simulink model "MicrogridControl"  (R2025b)
settings: Solver=VariableStepAuto  StartTime=0.0  StopTime=8  FixedStep=Ts  RelTol=1e-3
PreLoadFcn:
  | NormalOperation;
  | MicrogridControlParam;
undefined symbols (not defined in the file): base, bessModeInitial, bessSystem, bessVoltage, breakerStatus, DiscIntNeverNeededParam, ee_sli_rtmsupport, event, gcbh, generator, gflInverter, gfmInverter, Inertia, lineInductance, lineResistance, machine, plannedIsland, pmsm, powerLimit, powerQuality, PV, PVInverter, ref, resync, solar, solarInsolationChange, systemFrequency, Ts, windController, windSystem, windTurbine
libraries: nesl_utility x234, ee_lib x174, fl_lib x143, eeGeneralControl x137, simulink x78, eeTransforms x47, slpidlib x23, nesl_utility_internal x12, eePwmGenerator x9, eeSinusoidalMeasurementV2 x9, custom_lib x7, batteryecm_lib x6
(part 2 of 25)

== system MicrogridControl/BESS ==
  BusElementIn : Inport  PortName=InBus  Element=activePower
  BusElementIn1 : Inport  PortName=InBus  Element=reactivePower
  BusElementIn2 : Inport  PortName=InBus  Element=voltage
  BusElementIn3 : Inport  PortName=InBus  Element=frequency
  BusElementIn4 : Inport  PortName=InBus  Element=mode
  BusElementIn5 : Inport  PortName=InBus  Element=activePowerBESS1
  BESS Integrated : Subsystem  Variant=on  VariantControlMode=label  LabelModeActiveChoice=Detailed  mask(Battery Energy Storage System (BESS)){fidelity=Detailed, bessController=Grid Forming, plantRating=bessSystem.plantRating/2, Vac=bessSystem.Vac, frequency=bessSystem.frequency, iMaxPU=bessSystem.iMaxPU, efficiency=bessSystem.converterEfficiency, baseVoltageDC=bessSystem.Vdc, filterInductance=bessSystem.filterInductance, filterResistance=bessSystem.filterResistance, maxSOC=bessSystem.maxSOC, minSOC=bessSystem.minSOC, converterFidelity=Average, fSw=bessSystem.switchingFrequency, activeDroop=bessSystem.activeDroop, reactiveDroop=bessSystem.reactiveDroop, maxSOCGFM=0.95, minSOCGFM=0.1, initialSOC=0.9, capacityType=Infinite, capacity=1000}
      mask prompts: fidelity "Modeling Option"; bessController "Operating Mode"; plantRating "BESS Rating (kW)"; Vac "Rated AC side voltage (phase-phase RMS) (V)"; frequency "Rated electrical frequency at AC side (Hz)"; iMaxPU "Maximum converter current (pu)"; efficiency "Converter Efficiency (%)"; baseVoltageDC "Voltage on DC side (V)"; filterInductance "Filter inductance (H)"; filterResistance "Filter series resistance (Ohm)"; maxSOC "Maximum  operating SOC"; minSOC "Minimum  operating SOC"; converterFidelity "Converter Fidelity"; fSw "Switching Frequency (kHz)"; activeDroop "Active droop"; reactiveDroop "Reactive droop"; maxSOCGFM "Maximum  operating SOC"; minSOCGFM "Minimum  operating SOC"; initialSOC "Initial SOC"; capacityType "Battery charge capacity"; capacity "Battery capacity (Ah)"
      mask help:
      | This block represents a flexible BESS that can be configured for different operational modes and modeling fidelities. It supports Grid-Following (GFL) and Grid-Forming (GFM) control strategies, along with two fidelity levels:
      |
      | Detailed – captures dynamic control loops and converter behavior for accurate transient analysis.
      | Simplified – optimized for faster simulations while preserving essential system characteristics.
      settings: CopyFcn=set_param(gcbh,'LinkStatus','none');
      mask Help: web('BESS.html')
      mask TypeOptions fidelity: Detailed | Simplified
      mask Callback fidelity:
      | component.mask.fidelitySelection;
      |     fidelity = get_param(gcb,'fidelity');
      |     mode = get_param(gcb,'bessController');
      |     maskObj = Simulink.Mask.get(gcb);
      |     allNames = {maskObj.Parameters.Name};
      |     effIdx = find(strcmp(allNames, 'efficiency'));
      |     tabGFL = maskObj.getDialogControl('cellSimplified');
      |     tabGFM = maskObj.getDialogControl('cellSimplifiedGFM');
      |     if strcmp(fidelity,'Simplified')
      |         maskObj.Parameters(effIdx).Visible = 'on';
      |         if strcmp(mode,'Grid Following')
      |             tabGFL.Visible = 'on';
      |             tabGFM.Visible = 'off';
      |         else
      |             tabGFL.Visible = 'off';
      |             tabGFM.Visible = 'on';
      |         end
      |     else
      |         maskObj.Parameters(effIdx).Visible = 'off';
      |         tabGFL.Visible = 'off';
      |         tabGFM.Visible = 'off';
      |     end
      mask TypeOptions bessController: Grid Following | Grid Forming
      mask Callback bessController:
      | fidelity = get_param(gcb,'fidelity');
      | mode = get_param(gcb,'bessController');
      | if strcmp(fidelity,'Detailed')
      |     component.mask.setBESSController;
      | else
      |     blockPath = [gcb,'/','Simplified'];
      |     component.mask.setBESSController(blockPath);
      | end
      | maskObj = Simulink.Mask.get(gcb);
      | tabGFL = maskObj.getDialogControl('cellSimplified');
      | tabGFM = maskObj.getDialogControl('cellSimplifiedGFM');
      | if strcmp(fidelity,'Simplified')
      |     if strcmp(mode,'Grid Following')
      |         tabGFL.Visible = 'on';
      |         tabGFM.Visible = 'off';
      |     else
      |         tabGFL.Visible = 'off';
      |         tabGFM.Visible = 'on';
      |     end
      | else
      |     tabGFL.Visible = 'off';
      |     tabGFM.Visible = 'off';
      | end
      mask TypeOptions converterFidelity: Detailed/BESS Plant/converterFidelity
      mask Callback converterFidelity:
      | blockPath = [gcb,'/','Detailed','/','BESS Plant','/','Converter'];
      | component.mask.converterFidelity(blockPath);
      mask TypeOptions fSw: Detailed/PV Plant & Controller/PV Plant/fSw
      mask TypeOptions initialSOC: Simplified/Grid Forming/initialSOC
      mask TypeOptions capacityType: Simplified/Grid Forming/capacityType
      mask Callback capacityType: component.mask.configureBatteryCapacity;
      mask TypeOptions capacity: Simplified/Grid Forming/capacity
      mask DialogControl generalDetailed Prompt: General
      mask DialogControl cellDetailed Prompt: Battery
      mask DialogControl configureBattery Prompt: Edit battery parameters
      mask DialogControl configureBattery Callback:
      | blockPath = [gcb,'/','Detailed','/','BESS Plant','/','Battery'] ;
      |     component.mask.openBlock(blockPath);
      mask DialogControl controllerDetailed Prompt: BESS Controller
      mask DialogControl configureBESSController Prompt: Edit BESS Controller
      mask DialogControl configureBESSController Callback:
      | controllerType = get_param(gcb,'bessController');
      |     blockPath = [gcb,'/','Detailed','/','BESS Controller','/',controllerType];
      |     component.mask.openBlock(blockPath);
      mask DialogControl cellSimplified Prompt: Battery
      mask DialogControl configureBatterySimplified Prompt: Edit battery parameters
      mask DialogControl configureBatterySimplified Callback:
      | mode = get_param(gcb,'bessController');
      |     blockPath = [gcb,'/','Simplified','/',mode,'/','Battery'] ;
      |     if strcmp(mode,'Grid Following')
      |         component.mask.openBlock(blockPath);
      |     end
      mask DialogControl converter Prompt: Converter
      mask DialogControl editConverter Prompt: Edit converter parameters
      mask DialogControl editConverter Callback:
      | converterFidelity = get_param(gcb,'converterFidelity');
      | blockPath = [gcb,'/','Detailed','/','BESS Plant','/','Converter','/',converterFidelity,'/','Converter'];
      | component.mask.openBlock(blockPath);
      mask DialogControl cellSimplifiedGFM Prompt: Battery
      mask Display: image('battery_detailed.png');
  BESS Integrated1 : Subsystem  Variant=on  VariantControlMode=label  LabelModeActiveChoice=Detailed  mask(Battery Energy Storage System (BESS)){fidelity=Detailed, bessController=Grid Forming, plantRating=bessSystem.plantRating/2, Vac=bessSystem.Vac, frequency=bessSystem.frequency, iMaxPU=bessSystem.iMaxPU, efficiency=bessSystem.converterEfficiency, baseVoltageDC=bessSystem.Vdc, filterInductance=bessSystem.filterInductance, filterResistance=bessSystem.filterResistance, maxSOC=bessSystem.maxSOC, minSOC=bessSystem.minSOC, converterFidelity=Average, fSw=bessSystem.switchingFrequency, activeDroop=bessSystem.activeDroop, reactiveDroop=bessSystem.reactiveDroop, maxSOCGFM=0.95, minSOCGFM=0.1, initialSOC=0.9, capacityType=Infinite, capacity=1000}
      mask prompts: fidelity "Modeling Option"; bessController "Operating Mode"; plantRating "BESS Rating (kW)"; Vac "Rated AC side voltage (phase-phase RMS) (V)"; frequency "Rated electrical frequency at AC side (Hz)"; iMaxPU "Maximum converter current (pu)"; efficiency "Converter Efficiency (%)"; baseVoltageDC "Voltage on DC side (V)"; filterInductance "Filter inductance (H)"; filterResistance "Filter series resistance (Ohm)"; maxSOC "Maximum  operating SOC"; minSOC "Minimum  operating SOC"; converterFidelity "Converter Fidelity"; fSw "Switching Frequency (kHz)"; activeDroop "Active droop"; reactiveDroop "Reactive droop"; maxSOCGFM "Maximum  operating SOC"; minSOCGFM "Minimum  operating SOC"; initialSOC "Initial SOC"; capacityType "Battery charge capacity"; capacity "Battery capacity (Ah)"
      mask help:
      | This block represents a flexible BESS that can be configured for different operational modes and modeling fidelities. It supports Grid-Following (GFL) and Grid-Forming (GFM) control strategies, along with two fidelity levels:
      |
      | Detailed – captures dynamic control loops and converter behavior for accurate transient analysis.
      | Simplified – optimized for faster simulations while preserving essential system characteristics.
      settings: CopyFcn=set_param(gcbh,'LinkStatus','none');
      mask Help: web('BESS.html')
      mask TypeOptions fidelity: Detailed | Simplified
      mask Callback fidelity:
      | component.mask.fidelitySelection;
      |     fidelity = get_param(gcb,'fidelity');
      |     mode = get_param(gcb,'bessController');
      |     maskObj = Simulink.Mask.get(gcb);
      |     allNames = {maskObj.Parameters.Name};
      |     effIdx = find(strcmp(allNames, 'efficiency'));
      |     tabGFL = maskObj.getDialogControl('cellSimplified');
      |     tabGFM = maskObj.getDialogControl('cellSimplifiedGFM');
      |     if strcmp(fidelity,'Simplified')
      |         maskObj.Parameters(effIdx).Visible = 'on';
      |         if strcmp(mode,'Grid Following')
      |             tabGFL.Visible = 'on';
      |             tabGFM.Visible = 'off';
      |         else
      |             tabGFL.Visible = 'off';
      |             tabGFM.Visible = 'on';
      |         end
      |     else
      |         maskObj.Parameters(effIdx).Visible = 'off';
      |         tabGFL.Visible = 'off';
      |         tabGFM.Visible = 'off';
      |     end
      mask TypeOptions bessController: Grid Following | Grid Forming
      mask Callback bessController:
      | fidelity = get_param(gcb,'fidelity');
      | mode = get_param(gcb,'bessController');
      | if strcmp(fidelity,'Detailed')
      |     component.mask.setBESSController;
      | else
      |     blockPath = [gcb,'/','Simplified'];
      |     component.mask.setBESSController(blockPath);
      | end
      | maskObj = Simulink.Mask.get(gcb);
      | tabGFL = maskObj.getDialogControl('cellSimplified');
      | tabGFM = maskObj.getDialogControl('cellSimplifiedGFM');
      | if strcmp(fidelity,'Simplified')
      |     if strcmp(mode,'Grid Following')
      |         tabGFL.Visible = 'on';
      |         tabGFM.Visible = 'off';
      |     else
      |         tabGFL.Visible = 'off';
      |         tabGFM.Visible = 'on';
      |     end
      | else
      |     tabGFL.Visible = 'off';
      |     tabGFM.Visible = 'off';
      | end
      mask TypeOptions converterFidelity: Detailed/BESS Plant/converterFidelity
      mask Callback converterFidelity:
      | blockPath = [gcb,'/','Detailed','/','BESS Plant','/','Converter'];
      | component.mask.converterFidelity(blockPath);
      mask TypeOptions fSw: Detailed/PV Plant & Controller/PV Plant/fSw
      mask TypeOptions initialSOC: Simplified/Grid Forming/initialSOC
      mask TypeOptions capacityType: Simplified/Grid Forming/capacityType
      mask Callback capacityType: component.mask.configureBatteryCapacity;
      mask TypeOptions capacity: Simplified/Grid Forming/capacity
      mask DialogControl generalDetailed Prompt: General
      mask DialogControl cellDetailed Prompt: Battery
      mask DialogControl configureBattery Prompt: Edit battery parameters
      mask DialogControl configureBattery Callback:
      | blockPath = [gcb,'/','Detailed','/','BESS Plant','/','Battery'] ;
      |     component.mask.openBlock(blockPath);
      mask DialogControl controllerDetailed Prompt: BESS Controller
      mask DialogControl configureBESSController Prompt: Edit BESS Controller
      mask DialogControl configureBESSController Callback:
      | controllerType = get_param(gcb,'bessController');
      |     blockPath = [gcb,'/','Detailed','/','BESS Controller','/',controllerType];
      |     component.mask.openBlock(blockPath);
      mask DialogControl cellSimplified Prompt: Battery
      mask DialogControl configureBatterySimplified Prompt: Edit battery parameters
      mask DialogControl configureBatterySimplified Callback:
      | mode = get_param(gcb,'bessController');
      |     blockPath = [gcb,'/','Simplified','/',mode,'/','Battery'] ;
      |     if strcmp(mode,'Grid Following')
      |         component.mask.openBlock(blockPath);
      |     end
      mask DialogControl converter Prompt: Converter
      mask DialogControl editConverter Prompt: Edit converter parameters
      mask DialogControl editConverter Callback:
      | converterFidelity = get_param(gcb,'converterFidelity');
      | blockPath = [gcb,'/','Detailed','/','BESS Plant','/','Converter','/',converterFidelity,'/','Converter'];
      | component.mask.openBlock(blockPath);
      mask DialogControl cellSimplifiedGFM Prompt: Battery
      mask Display: image('battery_detailed.png');
  BESS Integrated3 : Subsystem  Variant=on  VariantControlMode=label  LabelModeActiveChoice=Detailed  mask(Battery Energy Storage System (BESS)){fidelity=Detailed, bessController=Grid Forming, plantRating=bessSystem.plantRating*1.5, Vac=bessSystem.Vac, frequency=bessSystem.frequency, iMaxPU=bessSystem.iMaxPU, efficiency=bessSystem.converterEfficiency, baseVoltageDC=bessSystem.Vdc, filterInductance=bessSystem.filterInductance, filterResistance=bessSystem.filterResistance, maxSOC=bessSystem.maxSOC, minSOC=bessSystem.minSOC, converterFidelity=Average, fSw=bessSystem.switchingFrequency, activeDroop=bessSystem.activeDroop, reactiveDroop=bessSystem.reactiveDroop, maxSOCGFM=0.95, minSOCGFM=0.1, initialSOC=0.9, capacityType=Infinite, capacity=1000}
      mask prompts: fidelity "Modeling Option"; bessController "Operating Mode"; plantRating "BESS Rating (kW)"; Vac "Rated AC side voltage (phase-phase RMS) (V)"; frequency "Rated electrical frequency at AC side (Hz)"; iMaxPU "Maximum converter current (pu)"; efficiency "Converter Efficiency (%)"; baseVoltageDC "Voltage on DC side (V)"; filterInductance "Filter inductance (H)"; filterResistance "Filter series resistance (Ohm)"; maxSOC "Maximum  operating SOC"; minSOC "Minimum  operating SOC"; converterFidelity "Converter Fidelity"; fSw "Switching Frequency (kHz)"; activeDroop "Active droop"; reactiveDroop "Reactive droop"; maxSOCGFM "Maximum  operating SOC"; minSOCGFM "Minimum  operating SOC"; initialSOC "Initial SOC"; capacityType "Battery charge capacity"; capacity "Battery capacity (Ah)"
      mask help:
      | This block represents a flexible BESS that can be configured for different operational modes and modeling fidelities. It supports Grid-Following (GFL) and Grid-Forming (GFM) control strategies, along with two fidelity levels:
      |
      | Detailed – captures dynamic control loops and converter behavior for accurate transient analysis.
      | Simplified – optimized for faster simulations while preserving essential system characteristics.
      settings: CopyFcn=set_param(gcbh,'LinkStatus','none');
      mask Help: web('BESS.html')
      mask TypeOptions fidelity: Detailed | Simplified
      mask Callback fidelity:
      | component.mask.fidelitySelection;
      |     fidelity = get_param(gcb,'fidelity');
      |     mode = get_param(gcb,'bessController');
      |     maskObj = Simulink.Mask.get(gcb);
      |     allNames = {maskObj.Parameters.Name};
      |     effIdx = find(strcmp(allNames, 'efficiency'));
      |     tabGFL = maskObj.getDialogControl('cellSimplified');
      |     tabGFM = maskObj.getDialogControl('cellSimplifiedGFM');
      |     if strcmp(fidelity,'Simplified')
      |         maskObj.Parameters(effIdx).Visible = 'on';
      |         if strcmp(mode,'Grid Following')
      |             tabGFL.Visible = 'on';
      |             tabGFM.Visible = 'off';
      |         else
      |             tabGFL.Visible = 'off';
      |             tabGFM.Visible = 'on';
      |         end
      |     else
      |         maskObj.Parameters(effIdx).Visible = 'off';
      |         tabGFL.Visible = 'off';
      |         tabGFM.Visible = 'off';
      |     end
      mask TypeOptions bessController: Grid Following | Grid Forming
      mask Callback bessController:
      | fidelity = get_param(gcb,'fidelity');
      | mode = get_param(gcb,'bessController');
      | if strcmp(fidelity,'Detailed')
      |     component.mask.setBESSController;
      | else
      |     blockPath = [gcb,'/','Simplified'];
      |     component.mask.setBESSController(blockPath);
      | end
      | maskObj = Simulink.Mask.get(gcb);
      | tabGFL = maskObj.getDialogControl('cellSimplified');
      | tabGFM = maskObj.getDialogControl('cellSimplifiedGFM');
      | if strcmp(fidelity,'Simplified')
      |     if strcmp(mode,'Grid Following')
      |         tabGFL.Visible = 'on';
      |         tabGFM.Visible = 'off';
      |     else
      |         tabGFL.Visible = 'off';
      |         tabGFM.Visible = 'on';
      |     end
      | else
      |     tabGFL.Visible = 'off';
      |     tabGFM.Visible = 'off';
      | end
      mask TypeOptions converterFidelity: Detailed/BESS Plant/converterFidelity
      mask Callback converterFidelity:
      | blockPath = [gcb,'/','Detailed','/','BESS Plant','/','Converter'];
      | component.mask.converterFidelity(blockPath);
      mask TypeOptions fSw: Detailed/PV Plant & Controller/PV Plant/fSw
      mask TypeOptions initialSOC: Simplified/Grid Forming/initialSOC
      mask TypeOptions capacityType: Simplified/Grid Forming/capacityType
      mask Callback capacityType: component.mask.configureBatteryCapacity;
      mask TypeOptions capacity: Simplified/Grid Forming/capacity
      mask DialogControl generalDetailed Prompt: General
      mask DialogControl cellDetailed Prompt: Battery
      mask DialogControl configureBattery Prompt: Edit battery parameters
      mask DialogControl configureBattery Callback:
      | blockPath = [gcb,'/','Detailed','/','BESS Plant','/','Battery'] ;
      |     component.mask.openBlock(blockPath);
      mask DialogControl controllerDetailed Prompt: BESS Controller
      mask DialogControl configureBESSController Prompt: Edit BESS Controller
      mask DialogControl configureBESSController Callback:
      | controllerType = get_param(gcb,'bessController');
      |     blockPath = [gcb,'/','Detailed','/','BESS Controller','/',controllerType];
      |     component.mask.openBlock(blockPath);
      mask DialogControl cellSimplified Prompt: Battery
      mask DialogControl configureBatterySimplified Prompt: Edit battery parameters
      mask DialogControl configureBatterySimplified Callback:
      | mode = get_param(gcb,'bessController');
      |     blockPath = [gcb,'/','Simplified','/',mode,'/','Battery'] ;
      |     if strcmp(mode,'Grid Following')
      |         component.mask.openBlock(blockPath);
      |     end
      mask DialogControl converter Prompt: Converter
      mask DialogControl editConverter Prompt: Edit converter parameters
      mask DialogControl editConverter Callback:
      | converterFidelity = get_param(gcb,'converterFidelity');
      | blockPath = [gcb,'/','Detailed','/','BESS Plant','/','Converter','/',converterFidelity,'/','Converter'];
      | component.mask.openBlock(blockPath);
      mask DialogControl cellSimplifiedGFM Prompt: Battery
      mask Display: image('battery_detailed.png');
  Bus Selector : BusSelector  OutputSignals=activePower,reactivePower
  Bus Selector1 : BusSelector  OutputSignals=activePower,reactivePower
  Bus Selector2 : BusSelector  OutputSignals=activePower,reactivePower
  Constant : Constant
  Constant1 : Constant
  Constant3 : Constant  Value=ref.QBESS1MW
  Constant4 : Constant
  Constant5 : Constant  Value=0
  Constant7 : Constant  Value=0
  Delay : Delay  DelayLength=100  InitialCondition=bessModeInitial  InputProcessing=Columns as channels (frame based)
  Gain1 : Gain
  Rate Transition : RateTransition  Deterministic=off  OutPortSampleTime=Ts
  Rate Transition1 : RateTransition  OutPortSampleTime=Ts
  Rate Transition2 : RateTransition  Deterministic=off  OutPortSampleTime=Ts
  Rate Transition3 : RateTransition  OutPortSampleTime=Ts
  Scope2 : Scope  NumInputPorts=2
      settings: ActiveDisplayYMinimum=-0.28740391792348163  ActiveDisplayYMaximum=0.22078217074426204  DataLoggingVariableName=ScopeData53
  Scope3 : Scope  NumInputPorts=2
      settings: ActiveDisplayYMinimum=-0.88278351750877571  ActiveDisplayYMaximum=1.6943513796670802  DataLoggingVariableName=ScopeData54
  Scope4 : Scope  NumInputPorts=2
      settings: ActiveDisplayYMinimum=-0.88286408189414312  ActiveDisplayYMaximum=1.6939099105793236  DataLoggingVariableName=ScopeData55
  Transformer : Subsystem  Variant=on  VariantControlMode=label  LabelModeActiveChoice=Detailed  mask{fidelity=Detailed}
      mask prompts: fidelity "Modeling Option"
      mask TypeOptions fidelity: Detailed | Simplified
      mask Callback fidelity:
      | choice = get_param(gcb,'fidelity');
      | switch choice
      |     case 'Detailed'
      |         set_param(gcb, 'LabelModeActiveChoice', 'Detailed');
      |     case 'Simplified'
      |          set_param(gcb, 'LabelModeActiveChoice', 'Simplified');
      |     otherwise
      |         disp('Choose proper variant');
      | end
  Transformer1 : Subsystem  Variant=on  VariantControlMode=label  LabelModeActiveChoice=Detailed  mask{fidelity=Detailed}
      mask prompts: fidelity "Modeling Option"
      mask TypeOptions fidelity: Detailed | Simplified
      mask Callback fidelity:
      | choice = get_param(gcb,'fidelity');
      | switch choice
      |     case 'Detailed'
      |         set_param(gcb, 'LabelModeActiveChoice', 'Detailed');
      |     case 'Simplified'
      |          set_param(gcb, 'LabelModeActiveChoice', 'Simplified');
      |     otherwise
      |         disp('Choose proper variant');
      | end
  Transformer3 : Subsystem  Variant=on  VariantControlMode=label  LabelModeActiveChoice=Detailed  mask{fidelity=Detailed}
      mask prompts: fidelity "Modeling Option"
      mask TypeOptions fidelity: Detailed | Simplified
      mask Callback fidelity:
      | choice = get_param(gcb,'fidelity');
      | switch choice
      |     case 'Detailed'
      |         set_param(gcb, 'LabelModeActiveChoice', 'Detailed');
      |     case 'Simplified'
      |          set_param(gcb, 'LabelModeActiveChoice', 'Simplified');
      |     otherwise
      |         disp('Choose proper variant');
      | end
  ~ : PMIOPort  Side=Left
  wires:
  Constant1/1 -> BESS Integrated/2(FRef), BESS Integrated1/2(FRef)
  Constant/1 -> BESS Integrated/1(VRef), BESS Integrated1/1(VRef)
  Constant5/1 -> BESS Integrated/6(Reset), BESS Integrated1/6(Reset)
  Constant3/1 -> BESS Integrated/4(QRef), BESS Integrated1/4(QRef)
  BusElementIn/1 -> Rate Transition/1
  BusElementIn1/1 -> Rate Transition1/1
  BusElementIn2/1 -> Rate Transition2/1
  BusElementIn3/1 -> Rate Transition3/1
  Rate Transition2/1 -> BESS Integrated3/1(VRef)
  Rate Transition3/1 -> BESS Integrated3/2(FRef)
  BusElementIn4/1 -> Delay/1
  Constant7/1 -> BESS Integrated3/6(Reset)
  Delay/1 -> Gain1/1
  BESS Integrated3/1(Meas) -> Bus Selector/1
  Bus Selector/1 -> Scope2/1  "<activePower>"
  Bus Selector/2 -> Scope2/2  "<reactivePower>"
  BESS Integrated1/1(Meas) -> Bus Selector1/1
  BESS Integrated/1(Meas) -> Bus Selector2/1
  Bus Selector1/2 -> Scope3/2  "<reactivePower>"
  Bus Selector1/1 -> Scope3/1  "<activePower>"
  Rate Transition/1 -> BESS Integrated3/3(PRef)
  Rate Transition1/1 -> BESS Integrated3/4(QRef)
  Bus Selector2/1 -> Scope4/1  "<activePower>"
  Bus Selector2/2 -> Scope4/2  "<reactivePower>"
  Constant4/1 -> BESS Integrated1/5(Mode), BESS Integrated/5(Mode)
  BusElementIn5/1 -> BESS Integrated1/3(PRef), BESS Integrated/3(PRef)
  Gain1/1 -> BESS Integrated3/5(Mode)
  connections:
  BESS Integrated/RConn1 -- Transformer/LConn1
  BESS Integrated1/RConn1 -- Transformer1/LConn1
  BESS Integrated3/RConn1 -- Transformer3/LConn1
  Transformer1/RConn1 -- Transformer3/RConn1 -- Transformer/RConn1 -- ~/RConn1

== system MicrogridControl/Control Room ==
  Constant1 : Constant  Value=ref.PBESS3MW%0.4  SampleTime=-1
  Constant2 : Constant  Value=0
  Constant3 : Constant  SampleTime=-1
  Constant4 : Constant  Value=ref.QBESS3MW%0.2  SampleTime=-1
  Constant5 : Constant  SampleTime=-1
  Constant6 : Constant  Value=0
  Constant7 : Constant  Commented=on  Value=0.45  SampleTime=-1
  Constant8 : Constant  Commented=on  Value=0.2  SampleTime=-1
  Data Type Conversion{3,5..7} (4 alike) : DataTypeConversion  OutDataTypeStr=boolean  SaturateOnIntegerOverflow=off  RndMeth=Floor
  PlannedIslandCommand : Step  Time=event.plannedIslanding  SampleTime=Ts
  Resynch Command : Step  Time=event.resynchronization  SampleTime=Ts
  Resynch Command1 : Step  Time=event.resynchronization  After=0  SampleTime=Ts
  Step13 : Step  Time=1000  After=-1  SampleTime=Ts
  Step16 : Step  Time=1000  SampleTime=Ts
  Step8 : Step  Time=1000  SampleTime=Ts
  Sum : Sum  Inputs=|++
  Out Bus Element5 : Outport  PortName=CtrlRm  Element=blackStart
  Out Bus Element4 : Outport  PortName=CtrlRm  Element=blackStartReset
  Out Bus Element19 : Outport  PortName=CtrlRm  Element=PowerCmd
  Out Bus Element20 : Outport  PortName=CtrlRm  Element=unplannedIslanding
  Out Bus Element22 : Outport  PortName=CtrlRm  Element=BESSReactivePower
  Out Bus Element18 : Outport  PortName=CtrlRm  Element=Resync
  Out Bus Element3 : Outport  PortName=CtrlRm  Element=FRef
  Out Bus Element6 : Outport  PortName=CtrlRm  Element=plannedIslanding
  Out Bus Element1 : Outport  PortName=CtrlRm  Element=QRef
  Out Bus Element2 : Outport  PortName=CtrlRm  Element=VRef
  Out Bus Element : Outport  PortName=CtrlRm  Element=PRef
  BusElementOut : Outport  PortName=CtrlRm  Element=BRKcontrol
  wires:
  Constant4/1 -> Out Bus Element1/1  "Reactive Power Setpoint"
  Data Type Conversion6/1 -> Out Bus Element18/1
  Step13/1 -> Sum/1  "Blackstart"
  Data Type Conversion7/1 -> Out Bus Element5/1
  Data Type Conversion3/1 -> Out Bus Element6/1
  Step8/1 -> Data Type Conversion7/1, Sum/2  "Blackstart"
  Constant5/1 -> Out Bus Element3/1  "Frequency Setpoint"
  Constant6/1 -> Out Bus Element22/1
  PlannedIslandCommand/1 -> Data Type Conversion3/1  "Planned Island_Command2"
  Resynch Command1/1 -> Out Bus Element19/1  "Power Tracking Command"
  Resynch Command/1 -> Data Type Conversion6/1  "Resynch_Command2"
  Constant1/1 -> Out Bus Element/1  "Active Power setpoint"
  Sum/1 -> Out Bus Element4/1
  Constant3/1 -> Out Bus Element2/1  "Voltage Setpoint"
  Step16/1 -> Data Type Conversion5/1  "VF mode"
  Data Type Conversion5/1 -> Out Bus Element20/1
  Constant2/1 -> BusElementOut/1

== system MicrogridControl/Domestic Load ==
  Circuit Breaker : Subsystem
  Electrical Reference1 : fl_lib/Electrical/Electrical Elements/Electrical Reference
  Electrical Reference2 : fl_lib/Electrical/Electrical Elements/Electrical Reference
  Load1 : ee_lib/Passive/RLC Assemblies/Wye-Connected Load  port_option=ee.enum.threePhasePort.composite  parameterization=ee.enum.rlc.parameterization.ratedpower  component_structure=ee.enum.rlc.structure.R  component_structure_PQ=ee.enum.rlc.structure.SeriesRL  R=1 Ohm  L=1e-3 H  C=1e-6 F  VRated=11000 V  FRated=systemFrequency Hz  P=7.5e6 W  Qpos=1e6 A*V  Qneg=-1e2 A*V  R_parasitic=1e-6 Ohm  G_parasitic=1e-6 1/Ohm  R_parasitic_PQ=1e-6 Ohm  G_parasitic_PQ=1e-6 1/Ohm  Vmag0=0 V  Vang0=0 deg  Freq0=systemFrequency Hz  IL_specify=off  IL_priority=High  IL=[0, 0, 0] A  IL_nominal_specify=off  IL_nominal_value=1  IL_nominal_unit=A  VC_specify=off  VC_priority=High  VC=[0, 0, 0] V  VC_nominal_specify=off  VC_nominal_value=1  VC_nominal_unit=V
  Load2 : ee_lib/Passive/RLC Assemblies/Wye-Connected Load  port_option=ee.enum.threePhasePort.composite  parameterization=ee.enum.rlc.parameterization.ratedpower  component_structure=ee.enum.rlc.structure.R  component_structure_PQ=ee.enum.rlc.structure.SeriesRL  R=1 Ohm  L=1e-3 H  C=1e-6 F  VRated=11000 V  FRated=systemFrequency Hz  P=500e3 W  Qpos=10e3 A*V  Qneg=-1e2 A*V  R_parasitic=1e-6 Ohm  G_parasitic=1e-6 1/Ohm  R_parasitic_PQ=1e-6 Ohm  G_parasitic_PQ=1e-6 1/Ohm  Vmag0=0 V  Vang0=0 deg  Freq0=systemFrequency Hz  IL_specify=off  IL_priority=High  IL=[0, 0, 0] A  IL_nominal_specify=off  IL_nominal_value=1  IL_nominal_unit=A  VC_specify=off  VC_priority=High  VC=[0, 0, 0] V  VC_nominal_specify=off  VC_nominal_value=1  VC_nominal_unit=V
  Step : Step  Time=breakerStatus.load  Before=1  After=0  SampleTime=0
  ~ : PMIOPort  Side=Left
  wires:
  Step/1 -> Circuit Breaker/1(BRK)
  connections:
  Electrical Reference1/LConn1 -- Load1/RConn1
  Load1/LConn1 -- Circuit Breaker/LConn1 -- ~/RConn1
  Load2/LConn1 -- Circuit Breaker/RConn1
  Electrical Reference2/LConn1 -- Load2/RConn1

== system MicrogridControl/Generator ==
  Constant : Constant
  Generator Integrated : Subsystem  Variant=on  VariantControlMode=label  LabelModeActiveChoice=Detailed  mask(Generator){fidelity=Detailed, genRating=generator.rating/5, Vac=generator.Vac, frequency=generator.frequency, polePairs=generator.polePairs, pu_speed_reference=machine.speedReference, droop_percentage=machine.droop, pu_load_reference_setpoint=machine.loadReference, T_G=machine.timeConstandGovernor, T_CH=machine.timeConstantPrimeMover, base_torque=machine.baseTorque/5, pu_torque0=machine.initialTorque*0}
      mask prompts: fidelity "Modeling Option"; genRating "Generator Rating (kW)"; Vac "Rated AC side voltage (phase-phase RMS) (V)"; frequency "Rated electrical frequency at AC side (Hz)"; polePairs "Number of pole pairs"; pu_speed_reference "Speed reference, (pu)"; droop_percentage "Percentage droop, (%)"; pu_load_reference_setpoint "Load reference setpoint, (pu)"; T_G "Time constant of governor, (s)"; T_CH "Time constant of main inlet volumes and steam chest, (s)"; base_torque "Base torque, (N*m)"; pu_torque0 "Initial torque, (pu)"
      mask help:
      | This block models a Generator. The detailed variant models AVR, Exciter, Prime mover, and Governer. The simplified variant is based on load torque and a constant field circuit current. Select simplified mode for faster simulation using fixed efficiency and rated power.
      |
      | Provide load reference as input
      settings: CopyFcn=set_param(gcbh,'LinkStatus','none');
      mask Help: web('Generator.html')
      mask TypeOptions fidelity: Detailed | Simplified
      mask Callback fidelity:
      | detailedTabs = {'generatorDetailed','exciterParam','governerParam',};
      |     simplifiedTabs = {'generatorSimplified'};
      |     component.mask.fidelitySelection(detailedTabs,simplifiedTabs);
      |     component.mask.fidelitySelection;
      mask TypeOptions pu_speed_reference:
      | Detailed/Governor and
      | Prime Mover
      | /pu_speed_reference
      mask TypeOptions droop_percentage:
      | Detailed/Governor and
      | Prime Mover
      | /droop_percentage
      mask TypeOptions pu_load_reference_setpoint:
      | Detailed/Governor and
      | Prime Mover
      | /pu_load_reference_setpoint
      mask TypeOptions T_G:
      | Detailed/Governor and
      | Prime Mover
      | /T_G
      mask TypeOptions T_CH:
      | Detailed/Governor and
      | Prime Mover
      | /T_CH
      mask TypeOptions base_torque:
      | Detailed/Governor and
      | Prime Mover
      | /base_torque
      mask TypeOptions pu_torque0:
      | Detailed/Governor and
      | Prime Mover
      | /pu_torque0
      mask DialogControl generalDetailed Prompt: General
      mask DialogControl editMachine Prompt: Edit machine parameters
      mask DialogControl editMachine Callback:
      | blockFidelity = get_param(gcb,'fidelity');
      |     blockPath = [gcb,'/',blockFidelity,'/','Machine'];
      |     component.mask.openBlock(blockPath);
      mask DialogControl editInertia Prompt: Edit inertia parameters
      mask DialogControl editInertia Callback:
      | blockPath = [gcb,'/','Detailed','/','Inertia'];
      |     component.mask.openBlock(blockPath);
      mask DialogControl exciterParam Prompt: Exciter
      mask DialogControl fieldParam Prompt: Edit field circuit parameters
      mask DialogControl fieldParam Callback:
      | blockPath = [gcb,'/','Detailed','/','AVR and Exciter','/','Exciter'];
      |     component.mask.openBlock(blockPath);
      mask DialogControl avrParam Prompt: Edit AVR parameters
      mask DialogControl avrParam Callback:
      | blockPath = [gcb,'/','Detailed','/','AVR and Exciter','/','AVR'];
      |     component.mask.openBlock(blockPath);
      mask DialogControl governerParam Prompt: Governer and Prime Mover
  RLC (Three-Phase)6 : ee_lib/Passive/RLC Assemblies/RLC (Three-Phase)  port_option=ee.enum.threePhasePort.composite  component_structure=ee.enum.rlc.structure.SeriesRL  R=1e-3 Ohm  L=0.8e-3%1e-3 H  C=1e-6 F  R_parasitic=0 Ohm  G_parasitic=0 1/Ohm  IL_specify=on  IL_priority=None  IL=[0, 0, 0] A  IL_nominal_specify=off  IL_nominal_value=1  IL_nominal_unit=A  VC_specify=off  VC_priority=High  VC=[0, 0, 0] V  VC_nominal_specify=off  VC_nominal_value=1  VC_nominal_unit=V
      settings: InternalSimscapePortConfiguration="{\"Bottom\":[],\"Left\":[{\"id\":\"N1\",\"label\":\"~1\",\"type\":\"foundation.electrical.three_phase\"}],\"Right\":[{\"id\":\"N2\",\"label\":\"~2\",\"type\":\"foundation.electrical.three_phase\"}],\"Top\":[]}"
  Transformer : Subsystem  Variant=on  VariantControlMode=label  LabelModeActiveChoice=Detailed  mask{fidelity=Detailed}
      mask prompts: fidelity "Modeling Option"
      mask TypeOptions fidelity: Detailed | Simplified
      mask Callback fidelity:
      | choice = get_param(gcb,'fidelity');
      | switch choice
      |     case 'Detailed'
      |         set_param(gcb, 'LabelModeActiveChoice', 'Detailed');
      |     case 'Simplified'
      |          set_param(gcb, 'LabelModeActiveChoice', 'Simplified');
      |     otherwise
      |         disp('Choose proper variant');
      | end
  ~ : PMIOPort  Side=Left
  wires:
  Constant/1 -> Generator Integrated/1(PRef)
  connections:
  RLC (Three-Phase)6/LConn1 -- Transformer/RConn1
  ~/RConn1 -- RLC (Three-Phase)6/RConn1
  Generator Integrated/RConn1 -- Transformer/LConn1

== system MicrogridControl/Microgrid Controller ==
  BusElementIn7 : Inport  PortName=CtrlRm  Element=PowerCmd
  Bus Element In : Inport  PortName=CtrlRm  Element=plannedIslanding
  Bus Element In2 : Inport  PortName=CtrlRm  Element=unplannedIslanding
  Bus Element In6 : Inport  PortName=CtrlRm  Element=BRKcontrol
  Bus Element In1 : Inport  PortName=CtrlRm  Element=Resync
  Bus Element In15 : Inport  PortName=CtrlRm  Element=blackStart
  Bus Element In4 : Inport  PortName=CtrlRm  Element=PRef
  Bus Element In5 : Inport  PortName=CtrlRm  Element=QRef
  BusElementIn5 : Inport  PortName=CtrlRm  Element=VRef
  BusElementIn6 : Inport  PortName=CtrlRm  Element=FRef
  BusElementIn : Inport  Port=2  PortName=Grid  Element=gridVoltage
  BusElementIn1 : Inport  Port=2  PortName=Grid  Element=PCCVoltage
  BusElementIn2 : Inport  Port=2  PortName=Grid  Element=P
  BusElementIn3 : Inport  Port=2  PortName=Grid  Element=Q
  Breaker Control : Subsystem  mask(Breaker Control){}
      mask help: Control breaker at PCC
  Bus Selector : BusSelector  OutputSignals=motorBreaker
  Constant : Constant  Value=0
  Constant1 : Constant  Value=0  OutDataTypeStr=boolean
  Microgrid Control Functions : Subsystem
  Microgrid Supervisory Control : Subsystem
  Rate Transition : RateTransition  OutPortSampleTime=1e-3
  Reference Generation : Subsystem
  Subsystem1 : Subsystem
  Brk : Outport
  ref : Outport  Port=2
  MotorBrk : Outport  Port=3
  wires:
  Breaker Control/1(BrK Ctrl) -> Brk/1, Microgrid Supervisory Control/10(BreakerStatus)
  BusElementIn2/1 -> Microgrid Control Functions/3(PCC Active Power)
  Bus Element In4/1 -> Reference Generation/4(Control Room PRef)
  BusElementIn/1 -> Subsystem1/1(Grid Voltage)
  Subsystem1/1(mPLL) -> Microgrid Supervisory Control/9(mPLL), Microgrid Control Functions/1(mPLL)
  Microgrid Supervisory Control/1(BrKControl) -> Breaker Control/1(BrKControl)
  [Status] -> Rate Transition/1
  Rate Transition/1 -> Reference Generation/9(Status)
  Bus Element In2/1 -> Microgrid Supervisory Control/6(UnplannedIslandingEnable)
  Reference Generation/1(ref) -> ref/1
  BusElementIn3/1 -> Microgrid Control Functions/4(PCC Reactive Power)
  BusElementIn1/1 -> Subsystem1/2(PCC Voltage)
  BusElementIn7/1 -> Reference Generation/8(Power Tracking)
  Bus Element In1/1 -> Microgrid Supervisory Control/4(Resync Enable)
  Bus Element In15/1 -> Microgrid Supervisory Control/7(BlackStart Enable)
  Bus Element In5/1 -> Reference Generation/5(Control Room QRef)
  BusElementIn6/1 -> Reference Generation/7(Control Room FRef)
  Bus Element In6/1 -> Breaker Control/2(CtrlRm BRK)
  Bus Element In/1 -> Microgrid Supervisory Control/5(PlannedIslandEnable)
  Constant1/1 -> Microgrid Supervisory Control/8(Blackout Status)
  Microgrid Supervisory Control/2(Status) -> Bus Selector/1, [Status]
  [Status] -> Microgrid Control Functions/5(Status)
  Constant/1 -> Microgrid Control Functions/2(BESS Reactive Power)
  BusElementIn5/1 -> Reference Generation/6(Control Room VRef)
  Microgrid Control Functions/1(Resync) -> Reference Generation/1(Resync)
  Microgrid Control Functions/2(PlannedIslanding) -> Reference Generation/2(Planned Islanding)
  Microgrid Control Functions/3(BlackStart) -> Reference Generation/3(BlackStart)
  Microgrid Control Functions/4(Resync Status) -> Microgrid Supervisory Control/1(Resync Status)
  Microgrid Control Functions/5(PlannedIsland Status) -> Microgrid Supervisory Control/2(PlannedIslanding Status)
  Microgrid Control Functions/6(BlackStart Status) -> Microgrid Supervisory Control/3(BlackStart Status)
  Bus Selector/1 -> MotorBrk/1  "<motorBreaker>"

== system MicrogridControl/Motor Load ==
  Input : Inport
  Circuit Breaker : Subsystem
  Delay : Delay  DelayLength=1  InitialCondition=breakerStatus.motorInitial
  Motor Loads : Subsystem
  Rate Transition : RateTransition  InitialCondition=breakerStatus.motorInitial  OutPortSampleTime=Ts
  ~ : PMIOPort  Side=Left
  wires:
  Input/1 -> Delay/1
  Rate Transition/1 -> Circuit Breaker/1(BRK)
  Delay/1 -> Rate Transition/1
  connections:
  Circuit Breaker/RConn1 -- Motor Loads/RConn1
  Circuit Breaker/LConn1 -- ~/RConn1

== system MicrogridControl/Results ==
  Bus Element In : Inport  PortName=Grid  Element=P
  BusElementIn : Inport  PortName=Grid  Element=Q
  Bus Element In2 : Inport  Port=2  PortName=BESS  Element=P
  BusElementIn1 : Inport  Port=2  PortName=BESS  Element=Q
  Bus Element In3 : Inport  Port=3  PortName=Wind  Element=P
  BusElementIn2 : Inport  Port=3  PortName=Wind  Element=Q
  Bus Element In1 : Inport  Port=4  PortName=Solar  Element=P
  BusElementIn3 : Inport  Port=4  PortName=Solar  Element=Q
  Bus Element In4 : Inport  Port=5  PortName=Generator  Element=P
  BusElementIn4 : Inport  Port=5  PortName=Generator  Element=Q
  Bus Element In5 : Inport  Port=6  PortName=Load  Element=P
  BusElementIn5 : Inport  Port=6  PortName=Load  Element=Q
  Mux : Mux  Inputs=6
  Mux1 : Mux  Inputs=6
  Power : Scope
      settings: ActiveDisplayYMinimum=-1.0733157557199045  ActiveDisplayYMaximum=11.28289096235352  YLabel=Active Power (MW)  DataLoggingVariableName=ScopeData11
  Reactive Power : Scope
      settings: ActiveDisplayYMinimum=-1.0527166703349433  ActiveDisplayYMaximum=1.451794431551988  YLabel=Active Power (MW)  DataLoggingVariableName=ScopeData31
  wires:
  Bus Element In/1 -> Mux/1  "Grid"
  Bus Element In2/1 -> Mux/2  "BESS"
  Bus Element In3/1 -> Mux/3  "Wind"
  Bus Element In1/1 -> Mux/4  "Solar"
  Bus Element In4/1 -> Mux/5  "Generator"
  Bus Element In5/1 -> Mux/6  "Load"
  Mux/1 -> Power/1
  BusElementIn/1 -> Mux1/1  "Grid"
  BusElementIn1/1 -> Mux1/2  "BESS"
  BusElementIn2/1 -> Mux1/3  "Wind"
  BusElementIn3/1 -> Mux1/4  "Solar"
  BusElementIn4/1 -> Mux1/5  "Generator"
  BusElementIn5/1 -> Mux1/6  "Load"
  Mux1/1 -> Reactive Power/1
